simulink model "OMAP"  (R2018b)
settings: Solver=FixedStepDiscrete  StartTime=0.0  StopTime=10.0  FixedStep=0.01  RelTol=1e-3
values from neighbouring files (symbols this model uses):
  Clb_ICADirect_LaneDisp_StateFive = Simulink.Parameter    [omap_ver_442.m]
  Clb_ICADirect_LaneDisp_StateFour = Simulink.Parameter    [omap_ver_442.m]
  Clb_ICADirect_LaneDisp_StateOne = Simulink.Parameter    [omap_ver_442.m]
  Clb_ICADirect_LaneDisp_StateThree = Simulink.Parameter    [omap_ver_442.m]
  Clb_ICADirect_LaneDisp_StateTwo = Simulink.Parameter    [omap_ver_442.m]
  Clb_ICADirect_LaneDisp_StateZero = Simulink.Parameter    [omap_ver_442.m]
  Clb_ICADirect_LaneDispSW = Simulink.Parameter    [omap_ver_442.m]
  Clb_ICADirect_TrnLghtsCom_Switch = Simulink.Parameter    [omap_ver_442.m]
  Clb_ICADirect_TrnLghtsCom_Value = Simulink.Parameter    [omap_ver_442.m]
  Clb_ICADirect_TrnLghtsCrtl_Inhb = Simulink.Parameter    [omap_ver_442.m]
  OMAP_ACCAEB_EMSESC_Decel = Simulink.Parameter    [omap_ver_442.m]
  OMAP_ACCFCW_IC_Decel = Simulink.Parameter    [omap_ver_442.m]
  OMAP_clb_ACC_RVVReqType = Simulink.Parameter    [omap_ver_442.m]
  OMAP_clb_ACC_RVVReqType_Switch = Simulink.Parameter    [omap_ver_442.m]
  OMAP_clb_ACCHeadwayDisplay = Simulink.Parameter    [omap_ver_442.m]
  OMAP_clb_ACCHeadwayDisplay_Switch = Simulink.Parameter    [omap_ver_442.m]
  OMAP_clb_ACCHeadwayIcon = Simulink.Parameter    [omap_ver_442.m]
  OMAP_clb_ACCHeadwayIcon_Switch = Simulink.Parameter    [omap_ver_442.m]
  OMAP_clb_ACCMessagePrompt = Simulink.Parameter    [omap_ver_442.m]
  OMAP_clb_ACCMessagePrompt_Switch = Simulink.Parameter    [omap_ver_442.m]
  OMAP_clb_ACCRequestEPB = Simulink.Parameter    [omap_ver_442.m]
  OMAP_clb_ACCRequestEPB_Switch = Simulink.Parameter    [omap_ver_442.m]
  OMAP_clb_ACCSetSpeed = Simulink.Parameter    [omap_ver_442.m]
  OMAP_clb_ACCSetSpeed_Switch = Simulink.Parameter    [omap_ver_442.m]
  OMAP_clb_ACCSetSpeedDis = Simulink.Parameter    [omap_ver_442.m]
  OMAP_clb_ACCSetSpeedDis_Switch = Simulink.Parameter    [omap_ver_442.m]
  OMAP_clb_ACCState = Simulink.Parameter    [omap_ver_442.m]
  OMAP_clb_ACCState_Switch = Simulink.Parameter    [omap_ver_442.m]
  OMAP_clb_ACCStatusIconDis = Simulink.Parameter    [omap_ver_442.m]
  OMAP_clb_ACCStatusIconDis_Switch = Simulink.Parameter    [omap_ver_442.m]
  OMAP_clb_ACCTorqueReq = Simulink.Parameter    [omap_ver_442.m]
  OMAP_clb_ACCTorqueReq_Switch = Simulink.Parameter    [omap_ver_442.m]
  OMAP_clb_ADAS_State = Simulink.Parameter    [omap_ver_442.m]
  OMAP_clb_ADAS_State_Switch = Simulink.Parameter    [omap_ver_442.m]
  OMAP_clb_AEBAlertReq = Simulink.Parameter    [omap_ver_442.m]
  OMAP_clb_AEBAlertReq_Switch = Simulink.Parameter    [omap_ver_442.m]
  OMAP_clb_AEBBrakingProg = Simulink.Parameter    [omap_ver_442.m]
  OMAP_clb_AEBBrakingProg_Switch = Simulink.Parameter    [omap_ver_442.m]
  OMAP_clb_AEBFaultStatus = Simulink.Parameter    [omap_ver_442.m]
  OMAP_clb_AEBFaultStatus_Switch = Simulink.Parameter    [omap_ver_442.m]
  OMAP_clb_AEBMassageDisp = Simulink.Parameter    [omap_ver_442.m]
  OMAP_clb_AEBMassageDisp_Switch = Simulink.Parameter    [omap_ver_442.m]
  OMAP_clb_AEBState = Simulink.Parameter    [omap_ver_442.m]
  OMAP_clb_AEBState_Switch = Simulink.Parameter    [omap_ver_442.m]
  OMAP_clb_AEBSwitchStatus = Simulink.Parameter    [omap_ver_442.m]
  OMAP_clb_AEBSwitchStatus_Switch = Simulink.Parameter    [omap_ver_442.m]
  OMAP_clb_BrakeRequest = Simulink.Parameter    [omap_ver_442.m]
  OMAP_clb_BrakeRequest_Switch = Simulink.Parameter    [omap_ver_442.m]
  OMAP_clb_DecelerationSet = Simulink.Parameter    [omap_ver_442.m]
  OMAP_clb_DecelerationSet_Switch = Simulink.Parameter    [omap_ver_442.m]
  OMAP_clb_DecelerationType = Simulink.Parameter    [omap_ver_442.m]
  OMAP_clb_DecelerationType_Switch = Simulink.Parameter    [omap_ver_442.m]
  OMAP_clb_DeclControlReq = Simulink.Parameter    [omap_ver_442.m]
  OMAP_clb_DeclControlReq_Switch = Simulink.Parameter    [omap_ver_442.m]
  OMAP_clb_DownorUpGearMinTime = Simulink.Parameter    [omap_ver_442.m]
  OMAP_clb_DownorUpGearMinTime_Switch = Simulink.Parameter    [omap_ver_442.m]
  OMAP_clb_ELKPopupMessage = Simulink.Parameter    [omap_ver_442.m]
  OMAP_clb_ELKPopupMessage_Switch = Simulink.Parameter    [omap_ver_442.m]
  OMAP_clb_ELKSts = Simulink.Parameter    [omap_ver_442.m]
  OMAP_clb_ELKSts_Switch = Simulink.Parameter    [omap_ver_442.m]
  OMAP_clb_ESAFaultSt = Simulink.Parameter    [omap_ver_442.m]
  OMAP_clb_ESAFaultSt_Switch = Simulink.Parameter    [omap_ver_442.m]
  OMAP_clb_ESARequest = Simulink.Parameter    [omap_ver_442.m]
  OMAP_clb_ESARequest_Switch = Simulink.Parameter    [omap_ver_442.m]
  OMAP_clb_ESAState = Simulink.Parameter    [omap_ver_442.m]
  OMAP_clb_ESAState_Switch = Simulink.Parameter    [omap_ver_442.m]
  OMAP_clb_ESATorqueReq = Simulink.Parameter    [omap_ver_442.m]
  OMAP_clb_ESATorqueReq_Switch = Simulink.Parameter    [omap_ver_442.m]
  OMAP_clb_ESCDriveOff = Simulink.Parameter    [omap_ver_442.m]
  OMAP_clb_ESCDriveOff_Switch = Simulink.Parameter    [omap_ver_442.m]
  OMAP_clb_ESCHoldReq = Simulink.Parameter    [omap_ver_442.m]
  OMAP_clb_ESCHoldReq_Switch = Simulink.Parameter    [omap_ver_442.m]
  OMAP_clb_Handsoffwarning = Simulink.Parameter    [omap_ver_442.m]
  OMAP_clb_Handsoffwarning_Switch = Simulink.Parameter    [omap_ver_442.m]
  OMAP_clb_HapticAlarmReq = Simulink.Parameter    [omap_ver_442.m]
  OMAP_clb_HapticAlarmReq_Switch = Simulink.Parameter    [omap_ver_442.m]
  OMAP_clb_HMIPopupMassage = Simulink.Parameter    [omap_ver_442.m]
  OMAP_clb_HMIPopupMassage_Switch = Simulink.Parameter    [omap_ver_442.m]
  OMAP_clb_HWAActionSts = Simulink.Parameter    [omap_ver_442.m]
  OMAP_clb_HWAActionSts_Switch = Simulink.Parameter    [omap_ver_442.m]
  OMAP_clb_HWAMode = Simulink.Parameter    [omap_ver_442.m]
  OMAP_clb_HWAMode_Switch = Simulink.Parameter    [omap_ver_442.m]
  OMAP_clb_HWATurnOnIdctr = Simulink.Parameter    [omap_ver_442.m]
  OMAP_clb_HWATurnOnIdctr_Switch = Simulink.Parameter    [omap_ver_442.m]
  OMAP_clb_ICAMassageDisp = Simulink.Parameter    [omap_ver_442.m]
  OMAP_clb_ICAMassageDisp_Switch = Simulink.Parameter    [omap_ver_442.m]
  OMAP_clb_ICAStatusIcon = Simulink.Parameter    [omap_ver_442.m]
  OMAP_clb_ICAStatusIcon_Switch = Simulink.Parameter    [omap_ver_442.m]
  OMAP_clb_ISLCDriverRemind = Simulink.Parameter    [omap_ver_442.m]
  OMAP_clb_ISLCDriverRemind_Switch = Simulink.Parameter    [omap_ver_442.m]
  OMAP_clb_ISLCState = Simulink.Parameter    [omap_ver_442.m]
  OMAP_clb_ISLCState_Switch = Simulink.Parameter    [omap_ver_442.m]
  OMAP_clb_JAFaultSt = Simulink.Parameter    [omap_ver_442.m]
  OMAP_clb_JAFaultSt_Switch = Simulink.Parameter    [omap_ver_442.m]
  OMAP_clb_LCAPopupMessage = Simulink.Parameter    [omap_ver_442.m]
  OMAP_clb_LCAPopupMessage_Switch = Simulink.Parameter    [omap_ver_442.m]
  OMAP_clb_LCAStatusDisplay = Simulink.Parameter    [omap_ver_442.m]
  OMAP_clb_LCAStatusDisplay_Switch = Simulink.Parameter    [omap_ver_442.m]
  OMAP_clb_LDWStatusDisplay = Simulink.Parameter    [omap_ver_442.m]
  OMAP_clb_LDWStatusDisplay_Switch = Simulink.Parameter    [omap_ver_442.m]
  OMAP_clb_LDWWarningSt = Simulink.Parameter    [omap_ver_442.m]
  OMAP_clb_LDWWarningSt_Switch = Simulink.Parameter    [omap_ver_442.m]
  OMAP_clb_LightControlValid = Simulink.Parameter    [omap_ver_442.m]
  OMAP_clb_LightControlValid_Switch = Simulink.Parameter    [omap_ver_442.m]
  OMAP_clb_LKAActivation = Simulink.Parameter    [omap_ver_442.m]
  OMAP_clb_LKAActivation_Switch = Simulink.Parameter    [omap_ver_442.m]
  OMAP_clb_LKAAngleReq = Simulink.Parameter    [omap_ver_442.m]
  OMAP_clb_LKAAngleReq_Switch = Simulink.Parameter    [omap_ver_442.m]
  OMAP_clb_LKAMode = Simulink.Parameter    [omap_ver_442.m]
  OMAP_clb_LKAMode_Switch = Simulink.Parameter    [omap_ver_442.m]
  OMAP_clb_LKAorELK_CoolTime = Simulink.Parameter    [omap_ver_442.m]
  OMAP_clb_LKAState = Simulink.Parameter    [omap_ver_442.m]
  OMAP_clb_LKAState_Switch = Simulink.Parameter    [omap_ver_442.m]
  OMAP_clb_LKAStatusDisplay = Simulink.Parameter    [omap_ver_442.m]
  OMAP_clb_LKAStatusDisplay_Switch = Simulink.Parameter    [omap_ver_442.m]
  OMAP_clb_LKASwitchState = Simulink.Parameter    [omap_ver_442.m]
  OMAP_clb_LKASwitchState_Switch = Simulink.Parameter    [omap_ver_442.m]
  OMAP_clb_LKATorqFactReq = Simulink.Parameter    [omap_ver_442.m]
  OMAP_clb_LKATorqFactReq_Switch = Simulink.Parameter    [omap_ver_442.m]
  OMAP_clb_PrefillRequest = Simulink.Parameter    [omap_ver_442.m]
  ... (+36 more)
libraries: simulink x184, canmsglib x2
(part 10 of 14)

== system OMAP/Runnable_OMAP_10ms_sys/OMAP_Module/ICA_Direct_G59/ICA_Define/Subsystem1/Dspl ==
  note: 0是运动，1是静止
  note: 0 ：可以从降级回到正常，
      | 1 ：不可以从降级回到正常
  TxHndOff : Inport
  Dspl_stTkOvStChk : Inport  Port=2
  Dspl_facmL0Ql : Inport  Port=3
  Dspl_facmR0Ql : Inport  Port=4
  Dspl_stVehSty : Inport  Port=5
  Dspl_facmL0Type : Inport  Port=6
  Dspl_facmR0Type : Inport  Port=7
  Dspl_stTHState : Inport  Port=8
  Dspl_bsFromFMCMsg : Inport  Port=9
  Dspl_stTHFKeyState : Inport  Port=10
  DsplPrcs_CIb : Inport  Port=11
  Dspl_tfAddVocCmd : Inport  Port=12
  DsplPrcs_dDgrdIconWarnflag : Inport  Port=13
  DsplPrcs_stSWALimFlg : Inport  Port=14
  Dspl_stturn_lightState : Inport  Port=15
  Dspl_stTLC_ALCmodeSW : Inport  Port=16
  Dspl_stLC_SpdCndtFlg : Inport  Port=17
  Bus Selector5 : BusSelector  OutputSignals=TH_HMIClb_tiHndOffTxtWarnT_C,TH_HMIClb_tiDgrdVocWarnDurT_C,TH_HMIClb_tiHndOffVocWarnT_C,TH_HMIClb_tiTxtLimT_C,TH_HMIClb_tiDgrdIconWarnHiDurT_C,TH_HMIClb_tiDgrdIconWarnLoDurT_C,TH_HMIClb_tiSWALimFlgDetT_C,TH_HMIClb_tiCalcPer_C
  Data Type Conversion{,1..6} (7 alike) : DataTypeConversion  OutDataTypeStr=uint16
  DsplPrcs : Subsystem
  TimePrcs : Subsystem
  Dspl_stTxtDspl : Outport
  Dspl_stICAIcon : Outport  Port=2
  Dspl_stLaneDspl : Outport  Port=3
  Dspl_stL0DispType : Outport  Port=4
  Dspl_stR0DispType : Outport  Port=5
  Dspl_stVocDspl : Outport  Port=6
  Dspl_stHWAmode : Outport  Port=7
  Dspl_bsMon : Outport  Port=8
  wires:
  Dspl_stTHState/1 -> DsplPrcs/7(DsplPrcs_stTHState)
  Dspl_stTHFKeyState/1 -> DsplPrcs/9(DsplPrcs_stTHFKeyState)
  Dspl_bsFromFMCMsg/1 -> DsplPrcs/8(DsplPrcs_bsFromFMCMsg)
  Data Type Conversion/1 -> Dspl_stTxtDspl/1
  Data Type Conversion1/1 -> Dspl_stICAIcon/1
  Data Type Conversion2/1 -> Dspl_stLaneDspl/1
  DsplPrcs/6(DsplPrcs_stVocDspl) -> Data Type Conversion5/1
  DsplPrcs/1(DsplPrcs_stTxtDspl) -> Data Type Conversion/1
  DsplPrcs/2(DsplPrcs_stICAIcon) -> Data Type Conversion1/1
  Data Type Conversion5/1 -> Dspl_stVocDspl/1
  DsplPrcs/8(DsplPrcs_bsMon) -> Dspl_bsMon/1
  DsplPrcs_CIb/1 -> Bus Selector5/1
  TimePrcs/2(TimePrcs_dDgrdVocWarnDurnum) -> DsplPrcs/18(DsplPrcs_dDgrdVocWarnDurnum)
  TimePrcs/3(TimePrcs_dHndOffVocWarnnum) -> DsplPrcs/19(DsplPrcs_dHndOffVocWarnnum)
  TimePrcs/1(TimePrcs_dHndOffTxtWarnnum) -> DsplPrcs/17(DsplPrcs_dHndOffTxtWarnnum)
  TimePrcs/4(TimePrcs_dTxtLimnum) -> DsplPrcs/20(DsplPrcs_dTxtLimnum)
  Bus Selector5/3 -> TimePrcs/3(TimePrcs_tiHndOffVocWarnT_C)  "<TH_HMIClb_tiHndOffVocWarnT_C>"
  Bus Selector5/8 -> TimePrcs/8(TimePrcs_tiCalcPer_C)  "<TH_HMIClb_tiCalcPer_C>"
  Bus Selector5/4 -> TimePrcs/4(TimePrcs_tiTxtLimT_C)  "<TH_HMIClb_tiTxtLimT_C>"
  Bus Selector5/1 -> TimePrcs/1(TimePrcs_tiHndOffTxtWarnT_C)  "<TH_HMIClb_tiHndOffTxtWarnT_C>"
  Bus Selector5/2 -> TimePrcs/2(TimePrcs_tiDgrdVocWarnDurT_C)  "<TH_HMIClb_tiDgrdVocWarnDurT_C>"
  TxHndOff/1 -> DsplPrcs/1(DsplPrcs_stStWhlHld)
  Dspl_facmL0Ql/1 -> DsplPrcs/3(DsplPrcs_facmL0Ql)
  Dspl_facmR0Ql/1 -> DsplPrcs/4(DsplPrcs_facmR0Ql)
  Dspl_stVehSty/1 -> DsplPrcs/10(DsplPrcs_stVehSty)
  Dspl_tfAddVocCmd/1 -> DsplPrcs/11(DsplPrcs_tfAddVocCmd)
  TimePrcs/5(TimePrcs_dDgrdIconWarnHiDurnum) -> DsplPrcs/21(DsplPrcs_dDgrdIconWarnHiDurnum)
  TimePrcs/6(TimePrcs_dDgrdIconWarnLoDurnum) -> DsplPrcs/22(DsplPrcs_dDgrdIconWarnLoDurnum)
  Bus Selector5/5 -> TimePrcs/5(TimePrcs_tiDgrdIconWarnHiDurT_C)  "<TH_HMIClb_tiDgrdIconWarnHiDurT_C>"
  Bus Selector5/6 -> TimePrcs/6(TimePrcs_tiDgrdIconWarnLoDurT_C)  "<TH_HMIClb_tiDgrdIconWarnLoDurT_C>"
  DsplPrcs_dDgrdIconWarnflag/1 -> DsplPrcs/13(DsplPrcs_dDgrdIconWarnflag)
  DsplPrcs_stSWALimFlg/1 -> DsplPrcs/12(DsplPrcs_stSWALimFlg)
  Bus Selector5/7 -> TimePrcs/7(TimePrcs_tiSWALimFlgDetT_C)  "<TH_HMIClb_tiSWALimFlgDetT_C>"
  TimePrcs/7(TimePrcs_tiSWALimFlgDetnum) -> DsplPrcs/23(DsplPrcs_tiSWALimFlgDetnum)
  Dspl_stTkOvStChk/1 -> DsplPrcs/2(DsplPrcs_stTkOvStChk)
  Dspl_facmL0Type/1 -> DsplPrcs/5(DsplPrcs_facmL0Type)
  Dspl_facmR0Type/1 -> DsplPrcs/6(DsplPrcs_facmR0Type)
  Data Type Conversion3/1 -> Dspl_stL0DispType/1
  Data Type Conversion4/1 -> Dspl_stR0DispType/1
  DsplPrcs/3(DsplPrcs_stLaneDspl) -> Data Type Conversion2/1
  DsplPrcs/4(DsplPrcs_stL0DispType) -> Data Type Conversion3/1
  DsplPrcs/5(DsplPrcs_stR0DispType) -> Data Type Conversion4/1
  Dspl_stturn_lightState/1 -> DsplPrcs/14(DsplPrcs_stturn_lightState)
  Dspl_stTLC_ALCmodeSW/1 -> DsplPrcs/15(DsplPrcs_stTLC_ALCmodeSW)
  Dspl_stLC_SpdCndtFlg/1 -> DsplPrcs/16(DsplPrcs_stLC_SpdCndtFlg)
  DsplPrcs/7(DsplPrcs_stHWAmode) -> Data Type Conversion6/1
  Data Type Conversion6/1 -> Dspl_stHWAmode/1

== system OMAP/Runnable_OMAP_10ms_sys/OMAP_Module/ICA_Direct_G59/ICA_Define/Subsystem1/Subsystem ==
  Vehicle_Line_Display_Org : Inport
  LCRMode : Inport  Port=2
  High_Time : Inport  Port=3
  Low_Time : Inport  Port=4
  ISA_Value : Inport  Port=5
  ISA_Type : Inport  Port=6
  THMode : Inport  Port=7
  LC_Scene : Inport  Port=8
  Compare To Constant : simulink/Logic and Bit Operations/Compare To Constant  relop===  const=uint16(4)  OutDataTypeStr=boolean
  Compare To Constant1 : simulink/Logic and Bit Operations/Compare To Constant  relop===  const=uint16(2)  OutDataTypeStr=boolean
  Compare To Constant2 : simulink/Logic and Bit Operations/Compare To Constant  relop===  const=uint16(3)  OutDataTypeStr=boolean
  Constant4 : Constant  Value=0  OutDataTypeStr=uint16
  Constant5 : Constant  Value=0  OutDataTypeStr=uint16
  Constant6 : Constant  Value=0  OutDataTypeStr=uint16
  Data Type Conversion : DataTypeConversion  OutDataTypeStr=uint16
  Data Type Conversion1 : DataTypeConversion  OutDataTypeStr=uint16
  Gain : Gain  Gain=100
  Gain1 : Gain  Gain=100
  Logical Operator1 : Logic  Operator=OR  AllPortsSameDT=off  OutDataTypeStr=boolean
  MATLAB Function : MATLAB Function  TreatAsAtomicUnit=on
  Subsystem : Subsystem
  Switch{1..3,6} (4 alike) : Switch  Criteria=u2 > Threshold
  TSR_Version_Only_Sign_Type : Outport
  Vehicle_Line_Display : Outport  Port=2
  ISA Value : Outport  Port=3
  wires:
  Vehicle_Line_Display_Org/1 -> Vehicle_Line_Display/1
  Compare To Constant/1 -> Switch1/2
  MATLAB Function/1(TSR_Version_Only_Sign_Type) -> Switch2/1, Switch1/1
  Switch1/1 -> TSR_Version_Only_Sign_Type/1
  Subsystem/1(Signal) -> Switch2/2
  Constant5/1 -> Switch2/3
  Switch2/1 -> Switch3/1
  Constant6/1 -> Switch3/3
  Switch3/1 -> Switch1/3
  Logical Operator1/1 -> Switch3/2
  High_Time/1 -> Gain/1
  Low_Time/1 -> Gain1/1
  Gain/1 -> Data Type Conversion/1
  Gain1/1 -> Data Type Conversion1/1
  Data Type Conversion/1 -> Subsystem/1(HiDurnum)
  Data Type Conversion1/1 -> Subsystem/2(LoDurnum)
  THMode/1 -> [THMode], Compare To Constant/1
  ISA_Value/1 -> Switch6/1, Switch6/2
  Constant4/1 -> Switch6/3
  Switch6/1 -> ISA Value/1
  LC_Scene/1 -> MATLAB Function/2(LC_Scene)
  [THMode] -> MATLAB Function/1(TH_Mode)
  LCRMode/1 -> [stLCRMode], Compare To Constant1/1, Compare To Constant2/1
  Compare To Constant1/1 -> Logical Operator1/1
  Compare To Constant2/1 -> Logical Operator1/2
  [stLCRMode] -> MATLAB Function/3(stLCRMode)

== system OMAP/Runnable_OMAP_10ms_sys/OMAP_Module/ICA_Direct_G59/ICA_Define/Subsystem1/Subsystem1 ==
  note: 标定开关Calib_ICADirect_TrnLghtsCom_Switch默认值为1，走ICA_Direct内部判断
      | 标定值为0时，通过标定值Calib_ICADirect_TrnLghtsCom_Value来自主选择输出的值
  LCRMode : Inport
  Constant : Constant  OutDataTypeStr=uint16
  Constant1 : Constant  Value=2  OutDataTypeStr=uint16
  Constant2 : Constant  Value=0  OutDataTypeStr=uint16
  Constant3 : Constant  Value=Clb_ICADirect_TrnLghtsCom_Switch  OutDataTypeStr=uint16
  Constant4 : Constant  Value=Clb_ICADirect_TrnLghtsCom_Value  OutDataTypeStr=uint16
  Index Vector : MultiPortSwitch  DataPortOrder=Specify indices  DataPortIndices={2,3,0}  OutDataTypeStr=uint16
  Switch : Switch  Criteria=u2 > Threshold  OutDataTypeStr=uint16
  TurnLightsCmd : Outport
  wires:
  LCRMode/1 -> Index Vector/1
  Index Vector/1 -> Switch/1
  Constant/1 -> Index Vector/2
  Constant1/1 -> Index Vector/3
  Constant2/1 -> Index Vector/4
  Constant3/1 -> Switch/2
  Constant4/1 -> Switch/3
  Switch/1 -> TurnLightsCmd/1

== system OMAP/Runnable_OMAP_10ms_sys/OMAP_Module/ICA_Direct_G59/ICA_Define/TH_HMIClb/ISA_TYPE ==
  In2 : Inport
  Switch : Switch  Criteria=u2 ~= 0  OutDataTypeStr=uint16
  tmp : Constant  Value=0  OutDataTypeStr=uint16
  Out1 : Outport
  wires:
  In2/1 -> Switch/2, Switch/1
  Switch/1 -> Out1/1
  tmp/1 -> Switch/3

== system OMAP/Runnable_OMAP_10ms_sys/OMAP_Module/ICA_Direct_G59/ICA_Define/TH_HMIClb/ISA_Value ==
  In2 : Inport
  Switch : Switch  Criteria=u2 ~= 0  OutDataTypeStr=uint16
  tmp : Constant  Value=0  OutDataTypeStr=uint16
  Out1 : Outport
  wires:
  tmp/1 -> Switch/3
  Switch/1 -> Out1/1
  In2/1 -> Switch/1, Switch/2

== system OMAP/Runnable_OMAP_10ms_sys/OMAP_Module/ICA_Direct_G59/ICA_Define/TH_HMIClb/LCScene_tmp ==
  In2 : Inport
  Switch : Switch  Criteria=u2 ~= 0  OutDataTypeStr=uint16
  tmp : Constant  Value=0  OutDataTypeStr=uint16
  Out1 : Outport
  wires:
  In2/1 -> Switch/2, Switch/1
  Switch/1 -> Out1/1
  tmp/1 -> Switch/3

== system OMAP/Runnable_OMAP_10ms_sys/OMAP_Module/ICA_Direct_G59/ICA_Define/TH_HMIClb/Mode_tmp ==
  In2 : Inport
  Switch : Switch  Criteria=u2 ~= 0  OutDataTypeStr=uint16
  tmp : Constant  Value=0  OutDataTypeStr=uint16
  Out1 : Outport
  wires:
  tmp/1 -> Switch/3
  Switch/1 -> Out1/1
  In2/1 -> Switch/1, Switch/2

== system OMAP/Runnable_OMAP_10ms_sys/OMAP_Module/ICA_Direct_G59/ICA_Define/TH_HMIClb/TH_HMIClb_tiDgrdIconWarnHiDurT_C ==
  In2 : Inport
  Constant : Constant  Value=TH_HMIClb_tiDgrdIconWarnHiDurT_C  OutDataTypeStr=single
  Switch : Switch  Criteria=u2 ~= 0  OutDataTypeStr=single
  Out1 : Outport
  wires:
  Constant/1 -> Switch/3
  Switch/1 -> Out1/1
  In2/1 -> Switch/1, Switch/2

== system OMAP/Runnable_OMAP_10ms_sys/OMAP_Module/ICA_Direct_G59/ICA_Define/TH_HMIClb/TH_HMIClb_tiDgrdIconWarnLoDurT_C ==
  In2 : Inport
  Constant : Constant  Value=TH_HMIClb_tiDgrdIconWarnLoDurT_C  OutDataTypeStr=single
  Switch : Switch  Criteria=u2 ~= 0  OutDataTypeStr=single
  Out1 : Outport
  wires:
  In2/1 -> Switch/2, Switch/1
  Switch/1 -> Out1/1
  Constant/1 -> Switch/3

== system OMAP/Runnable_OMAP_10ms_sys/OMAP_Module/ICA_Direct_G59/ICA_Define/TH_HMIClb/TH_HMIClb_tiDgrdVocWarnDurT_C ==
  In2 : Inport
  Switch : Switch  Criteria=u2 ~= 0  OutDataTypeStr=single
  TH_MIN_SPEED_UPPER 1 : Constant  Value=TH_HMIClb_tiDgrdVocWarnDurT_C  OutDataTypeStr=single
  Out1 : Outport
  wires:
  In2/1 -> Switch/2, Switch/1
  Switch/1 -> Out1/1
  TH_MIN_SPEED_UPPER 1/1 -> Switch/3

== system OMAP/Runnable_OMAP_10ms_sys/OMAP_Module/ICA_Direct_G59/ICA_Define/TH_HMIClb/TH_HMIClb_tiHndOffTxtWarnT_C  ==
  In2 : Inport
  Switch : Switch  Criteria=u2 ~= 0  OutDataTypeStr=single
  TH_MIN_SPEED_UPPER 1 : Constant  Value=TH_HMIClb_tiHndOffTxtWarnT_C  OutDataTypeStr=single
  Out1 : Outport
  wires:
  In2/1 -> Switch/2, Switch/1
  Switch/1 -> Out1/1
  TH_MIN_SPEED_UPPER 1/1 -> Switch/3

== system OMAP/Runnable_OMAP_10ms_sys/OMAP_Module/ICA_Direct_G59/ICA_Define/TH_HMIClb/TH_HMIClb_tiHndOffVocWarnT_C ==
  In2 : Inport
  Switch : Switch  Criteria=u2 ~= 0  OutDataTypeStr=single
  TH_MIN_SPEED_UPPER 1 : Constant  Value=TH_HMIClb_tiHndOffVocWarnT_C  OutDataTypeStr=single
  Out1 : Outport
  wires:
  TH_MIN_SPEED_UPPER 1/1 -> Switch/3
  Switch/1 -> Out1/1
  In2/1 -> Switch/1, Switch/2

== system OMAP/Runnable_OMAP_10ms_sys/OMAP_Module/ICA_Direct_G59/ICA_Define/TH_HMIClb/TH_HMIClb_tiSWALimFlgDetT_C ==
  In2 : Inport
  Switch : Switch  Criteria=u2 ~= 0  OutDataTypeStr=single
  TH_HMIClb_tiSWALimFlgDetT_C : Constant  Value=TH_HMIClb_tiSWALimFlgDetT_C  OutDataTypeStr=single
  Out1 : Outport
  wires:
  TH_HMIClb_tiSWALimFlgDetT_C/1 -> Switch/3
  Switch/1 -> Out1/1
  In2/1 -> Switch/1, Switch/2

== system OMAP/Runnable_OMAP_10ms_sys/OMAP_Module/ICA_Direct_G59/ICA_Define/TH_HMIClb/TH_HMIClb_tiTxtLimT_C ==
  In2 : Inport
  Constant : Constant  Value=TH_HMIClb_tiTxtLimT_C  OutDataTypeStr=single
  Switch : Switch  Criteria=u2 ~= 0  OutDataTypeStr=single
  Out1 : Outport
  wires:
  In2/1 -> Switch/2, Switch/1
  Switch/1 -> Out1/1
  Constant/1 -> Switch/3

== system OMAP/Runnable_OMAP_10ms_sys/OMAP_Module/Subsystem/EMS_Arbitration/ACC//ICA_arb_AEB//JA/AEB_arb_JA ==
  note: 仲裁#1——AEB与JA
      | 1. JAEB/JACW无条件优先于FCW
      | 2. （在AEB系统内部，已经是AEB无条件优先于FCW）
      | 3. 对于AEB和JAEB/JACW，使能请求取或，请求值取较大者（若JA只开启报警、未开启制动，也就是只有JACW，那么制动请求值就很小，同样能符合此条效果）
      | 4. AEB_Alert能够标记减速发送者：2（AEB制动）、3（JA制动）
  Input_AEBS : Inport
  Input_JABS : Inport  Port=2
  Bus Creator3 : BusCreator  Inputs=5
  Bus Selector : BusSelector  OutputSignals=AEBSve_d_MDDdecRequest_convert,AEBSve_g_DecSetpoint_convert
  Bus Selector4 : BusSelector  OutputSignals=JABSve_d_DbMDDdecRequest_convert
  Compare To Constant1 : simulink/Logic and Bit Operations/Compare To Constant  relop=<  const=-2  OutDataTypeStr=boolean
  Compare To Constant4 : simulink/Logic and Bit Operations/Compare To Constant  relop===  const=1  OutDataTypeStr=boolean
  Compare To Constant5 : simulink/Logic and Bit Operations/Compare To Constant  relop===  const=1  OutDataTypeStr=boolean
  Compare To Constant6 : simulink/Logic and Bit Operations/Compare To Constant  relop=>=  const=-2  OutDataTypeStr=boolean
  Compare To Constant9 : simulink/Logic and Bit Operations/Compare To Constant  relop===  const=1  OutDataTypeStr=boolean
  Logical Operator : Logic  Operator=OR  AllPortsSameDT=off  OutDataTypeStr=boolean
  Logical Operator2 : Logic  AllPortsSameDT=off  OutDataTypeStr=boolean
  Logical Operator3 : Logic  AllPortsSameDT=off  OutDataTypeStr=boolean
  OMAPve_g_ACCTqReqNum1 : Constant  Value=-4000  OutDataTypeStr=single
  OMAPve_g_PotACCTqReqNum1 : Constant  Value=-4000  OutDataTypeStr=single
  OMAPve_g_TminUp_or_downGearNum2 : Constant  Value=0  OutDataTypeStr=single
  OMAPve_y_Powertrain_torquewheel_requestNum1 : Constant  Value=0  OutDataTypeStr=uint8
  OMAPve_y_stAcvTqWhlPTPotReqNum2 : Constant  Value=2  OutDataTypeStr=uint8
  Out1 : Outport
  Out2 : Outport  Port=2
  Out3 : Outport  Port=3
  wires:
  OMAPve_g_ACCTqReqNum1/1 -> Bus Creator3/2  "OMAPve_g_ACCTqReq_1"
  Compare To Constant9/1 -> Logical Operator2/1
  Input_AEBS/1 -> Bus Selector/1
  Bus Creator3/1 -> Out1/1
  OMAPve_g_PotACCTqReqNum1/1 -> Bus Creator3/1  "OMAPve_g_PotACCTqReq_1"
  OMAPve_g_TminUp_or_downGearNum2/1 -> Bus Creator3/4  "OMAPve_g_TminUp_or_downGear_1"
  Logical Operator2/1 -> Out3/1
  Compare To Constant4/1 -> Logical Operator/2
  OMAPve_y_stAcvTqWhlPTPotReqNum2/1 -> Bus Creator3/5  "OMAPve_y_stAcvTqWhlPTPotReq_1"
  Input_JABS/1 -> Bus Selector4/1
  Compare To Constant1/1 -> Logical Operator3/2
  OMAPve_y_Powertrain_torquewheel_requestNum1/1 -> Bus Creator3/3  "OMAPve_y_Powertrain_torquewheel_request_1"
  Bus Selector/1 -> Compare To Constant5/1, Compare To Constant9/1  "<AEBSve_d_MDDdecRequest_convert>"
  Bus Selector4/1 -> Compare To Constant4/1  "<JABSve_d_DbMDDdecRequest_convert>"
  Logical Operator/1 -> Out2/1
  Bus Selector/2 -> Compare To Constant1/1, Compare To Constant6/1  "<AEBSve_g_DecSetpoint_convert>"
  Compare To Constant6/1 -> Logical Operator2/2
  Logical Operator3/1 -> Logical Operator/1
  Compare To Constant5/1 -> Logical Operator3/1

== system OMAP/Runnable_OMAP_10ms_sys/OMAP_Module/Subsystem/EPS_Default_Arbitration/LKA_arb_ELK/Subsystem ==
  LKA_State : Inport
  ELK_State : Inport  Port=2
  In1 : Inport  Port=3
  Compare To Constant1 : simulink/Logic and Bit Operations/Compare To Constant  relop===  const=4  OutDataTypeStr=boolean
  Compare To Constant2 : simulink/Logic and Bit Operations/Compare To Constant  relop===  const=4  OutDataTypeStr=boolean
  Logical Operator : Logic  AllPortsSameDT=off  OutDataTypeStr=boolean
  Logical Operator1 : Logic  AllPortsSameDT=off  OutDataTypeStr=boolean
  Logical Operator2 : Logic  Operator=OR  AllPortsSameDT=off  OutDataTypeStr=boolean
  Logical Operator3 : Logic  Operator=OR  AllPortsSameDT=off  OutDataTypeStr=boolean
  Logical Operator4 : Logic  Operator=NOT  AllPortsSameDT=off  OutDataTypeStr=boolean
  Logical Operator5 : Logic  Operator=OR  AllPortsSameDT=off  OutDataTypeStr=boolean
  Memory : Memory
  Subsystem1 : Subsystem
  Subsystem2 : Subsystem
  Switch : Switch  Criteria=u2 > Threshold
  Out1 : Outport
  wires:
  Logical Operator1/1 -> Logical Operator5/2
  Logical Operator/1 -> Logical Operator5/1
  Logical Operator5/1 -> Switch/2, Memory/1
  Memory/1 -> Logical Operator1/2
  Subsystem2/1(Out1) -> Logical Operator1/1, Logical Operator2/2
  LKA_State/1 -> Compare To Constant2/1, Switch/3
  ELK_State/1 -> Switch/1, Compare To Constant1/1
  Compare To Constant1/1 -> Logical Operator2/1, Subsystem2/1(In1)
  Switch/1 -> Out1/1
  Compare To Constant2/1 -> Subsystem1/1(In1), Logical Operator3/1
  Subsystem1/1(Out1) -> Logical Operator3/2
  In1/1 -> Subsystem1/2(In2), Subsystem2/2(In2)
  Logical Operator2/1 -> Logical Operator/1
  Logical Operator3/1 -> Logical Operator4/1
  Logical Operator4/1 -> Logical Operator/2

== system OMAP/Runnable_OMAP_10ms_sys/OMAP_Module/Subsystem/EPS_Default_Arbitration/LKA_arb_ELK/Subsystem2 ==
  <LKASve_y_EPS_State_Control_convert> : Inport
  <OMAPve_y_General_state_of_LKA_function3F2_2> : Inport  Port=2
  Chart1 : Stateflow chart  TreatAsAtomicUnit=on
  Constant : Constant  Value=OMAP_clb_LKAorELK_CoolTime  OutDataTypeStr=single
  Subsystem1 : Subsystem
  state : Outport
  wires:
  Subsystem1/6(ELK_Active) -> Chart1/6(ELK_Active)
  Subsystem1/2(LKA_Down) -> Chart1/2(LKA_Down)
  Subsystem1/1(LKA_Up) -> Chart1/1(LKA_Up)
  Subsystem1/3(LKA_Active) -> Chart1/3(LKA_Active)
  <OMAPve_y_General_state_of_LKA_function3F2_2>/1 -> Subsystem1/2(ELK_State)
  <LKASve_y_EPS_State_Control_convert>/1 -> Subsystem1/1(LKA_State)
  Subsystem1/4(ELK_Up) -> Chart1/4(ELK_Up)
  Subsystem1/5(ELK_Down) -> Chart1/5(ELK_Down)
  Constant/1 -> Chart1/7(cool_time)
  Chart1/1(state) -> state/1

== system OMAP/Runnable_OMAP_10ms_sys/OMAP_Module/Subsystem/ESC_Arbitration/ACC//ICA_arb_AEB//JA/AEB_arb_JA ==
  note: 仲裁#1——AEB与JA
      | 1. JAEB/JACW无条件优先于FCW
      | 2. （在AEB系统内部，已经是AEB无条件优先于FCW）
      | 3. 对于AEB和JAEB/JACW，使能请求取或，请求值取较大者（若JA只开启报警、未开启制动，也就是只有JACW，那么制动请求值就很小，同样能符合此条效果）
      | 4. AEB_Alert能够标记减速发送者：2（AEB制动）、3（JA制动）
  note: 仲裁#11——AEB与JA的STATUS
      | 1. 关于对执行器发出的AEB_STATE——
      | 值7：对内，各自判断、各自对自己生效；对外OMAP发送：任一方fault就fault
      | 值6、5：对内，各自判断、各自对自己生效；对外OMAP发送：只以AEB的为准。特殊情况：如果AEB在3，但是JA在6、5，则对外发6、5
      | 值4：不用
      | 值3：对内，各自判断、各自对自己生效；对外OMAP发送：双方都inhibit才inhibit
      | 值2：不用
      | 值1：对内：JA可以不做。对外OMAP发送：只以AEB的为准
      | 值0：对内：JA可以不做。对外OMAP发送：只以AEB的为准
  note: 仲裁#8——AEB/FCW/JAEB/JACW与ELK
      | 1.AEB/FCW/JAEB/JACW无条件优先于ELK
  Input_AEBS : Inport
  Input_JABS : Inport  Port=2
  Input_ELKS : Inport  Port=3
  AEB/JA_arb_ELK : Subsystem
  AEB_arb_JA_STATUS : Subsystem
  Bus Creator : BusCreator  Inputs=5
  Bus Creator1 : BusCreator  Inputs=8
  Bus Selector5 : BusSelector  OutputSignals=AEBSve_d_FCWStatus_convert,AEBSve_d_functionFARCState_convert,AEBSve_d_AEBStatus_convert,AEBSve_d_Prefill_request_convert,AEBSve_d_AEBAlertReq_convert,AEBSve_d_HapticAlarm_convert,AEBSve_d_ESCDriveOff_convert,AEBSve_d_ESCHoldReq_convert,AEBSve_d_MDDdecType_convert,AEBSve_d_Braking_progress_convert,AEBSve_d_MDDdecRequest_convert,AEBSve_g_DecSetpoint_convert
  Bus Selector6 : BusSelector  OutputSignals=JABSve_g_DbDecSetpoint_convert,JABSve_d_DbMDDdecType_convert,JABSve_d_DbMDDdecRequest_convert,JABSve_d_DbPrefillReq_convert,JABSve_d_DbAlertReq_convert,JABSve_d_DbHapticAlarm_convert,JABSve_d_DbESCDriveOff_convert,JABSve_d_DbESCHoldReq_convert,JABSve_d_DbFunFARCSta_convert,JABSve_d_DbJACWStatus_convert
  Compare To Constant3 : simulink/Logic and Bit Operations/Compare To Constant  relop=<  const=-2  OutDataTypeStr=boolean
  Compare To Constant4 : simulink/Logic and Bit Operations/Compare To Constant  relop===  const=1  OutDataTypeStr=boolean
  Compare To Constant5 : simulink/Logic and Bit Operations/Compare To Constant  relop===  const=1  OutDataTypeStr=boolean
  Compare To Constant7 : simulink/Logic and Bit Operations/Compare To Constant  relop=>=  const=-2  OutDataTypeStr=boolean
  Compare To Constant8 : simulink/Logic and Bit Operations/Compare To Constant  relop===  const=1  OutDataTypeStr=boolean
  Data Type Conversion{1..2,9..10} (4 alike) : DataTypeConversion  OutDataTypeStr=uint8
  Logical Operator{,1,7..9} (5 alike) : Logic  Operator=OR  AllPortsSameDT=off  OutDataTypeStr=boolean
  Logical Operator2 : Logic  AllPortsSameDT=off  OutDataTypeStr=boolean
  Logical Operator5 : Logic  AllPortsSameDT=off  OutDataTypeStr=boolean
  OMAPve_y_ADAS_ACCRequestEPBNum : Constant  Value=0  OutDataTypeStr=uint8
  Relational Operator : RelationalOperator  Operator=<=  OutDataTypeStr=boolean  RndMeth=Simplest
  Switch10 : Switch  Criteria=u2 ~= 0  OutDataTypeStr=single
  Switch3 : Switch  Criteria=u2 ~= 0  OutDataTypeStr=uint8
  Switch6 : Switch  Criteria=u2 ~= 0  OutDataTypeStr=uint8
  Switch9 : Switch  Criteria=u2 ~= 0  OutDataTypeStr=uint8
  Terminator : Terminator
  Out1 : Outport
  Out2 : Outport  Port=2
  Out3 : Outport  Port=3
  Out4 : Outport  Port=4
  tag scope: ob_AEBarbJADecReq=global, ob_AEBarbJADecSet=global, ob_AEBarbJADecType=global
  wires:
  Bus Selector5/3 -> Terminator/1  "<AEBSve_d_AEBStatus_convert>"
  Bus Selector6/1 -> Switch10/3, Relational Operator/2  "<JABSve_g_DbDecSetpoint_convert>"
  Input_JABS/1 -> Bus Selector6/1
  Logical Operator7/1 -> Bus Creator/4  "OMAPve_y_Prefill_request_1"
  Bus Selector5/11 -> Compare To Constant4/1, Compare To Constant8/1, Switch9/1  "<AEBSve_d_MDDdecRequest_convert>"
  Bus Selector6/6 -> Logical Operator8/2  "<JABSve_d_DbHapticAlarm_convert>"
  Bus Creator/1 -> Out1/1
  Switch6/1 -> Bus Creator1/4, Data Type Conversion10/1  "OMAPve_y_AEB_Braking_progress_1"
  Bus Selector6/3 -> Compare To Constant5/1, Switch6/3, Switch9/3  "<JABSve_d_DbMDDdecRequest_convert>"
  Relational Operator/1 -> Switch3/2, Switch6/2, Switch9/2, Switch10/2
  Logical Operator2/1 -> Logical Operator/2
  Bus Selector5/10 -> Switch6/1  "<AEBSve_d_Braking_progress_convert>"
  Data Type Conversion10/1 -> Bus Creator1/5  "OMAPve_y_Decel_Request_1"
  Bus Selector5/12 -> Compare To Constant3/1, Compare To Constant7/1, Relational Operator/1, Switch10/1  "<AEBSve_g_DecSetpoint_convert>"
  Bus Selector5/9 -> Switch3/1  "<AEBSve_d_MDDdecType_convert>"
  AEB/JA_arb_ELK/1(Out1) -> Bus Creator/5  "OMAPve_y_Haptic_Alarm_1"
  Bus Creator1/1 -> Out2/1
  Bus Selector5/6 -> Logical Operator8/1  "<AEBSve_d_HapticAlarm_convert>"
  Input_AEBS/1 -> Bus Selector5/1
  Bus Selector6/2 -> Switch3/3  "<JABSve_d_DbMDDdecType_convert>"
  Bus Selector6/4 -> Logical Operator7/2  "<JABSve_d_DbPrefillReq_convert>"
  Bus Selector5/4 -> Logical Operator7/1  "<AEBSve_d_Prefill_request_convert>"
  Logical Operator/1 -> Out3/1
  Compare To Constant8/1 -> Logical Operator5/2
  Compare To Constant7/1 -> Logical Operator5/1
  Logical Operator5/1 -> Out4/1
  Compare To Constant5/1 -> Logical Operator/1
  Compare To Constant3/1 -> Logical Operator2/1
  Compare To Constant4/1 -> Logical Operator2/2
  AEB_arb_JA_STATUS/2(Out2) -> Bus Creator/2, Data Type Conversion9/1  "OMAPve_y_State_of_the_functionFARC_det_1"
  Data Type Conversion9/1 -> Bus Creator/3  "OMAPve_y_AEB_Status_1"
  AEB_arb_JA_STATUS/1(Out1) -> Bus Creator/1  "OMAPve_y_FCW_Status_1"
  Bus Selector5/1 -> AEB_arb_JA_STATUS/3(<AEBSve_d_FCWStatus_convert>)  "<AEBSve_d_FCWStatus_convert>"
  Bus Selector5/2 -> AEB_arb_JA_STATUS/4(<AEBSve_d_functionFARCState_convert>)  "<AEBSve_d_functionFARCState_convert>"
  Bus Selector6/9 -> AEB_arb_JA_STATUS/1(<JABSve_d_DbFunFARCSta_convert>)  "<JABSve_d_DbFunFARCSta_convert>"
  Bus Selector6/10 -> AEB_arb_JA_STATUS/2(<JABSve_d_DbJACWStatus_convert>)  "<JABSve_d_DbJACWStatus_convert>"
  Input_ELKS/1 -> AEB/JA_arb_ELK/1(Input_ELKS)
  Logical Operator8/1 -> AEB/JA_arb_ELK/4(AEB+JA_Haptic)
  Bus Selector5/5 -> AEB/JA_arb_ELK/2(AEB_Alert)  "<AEBSve_d_AEBAlertReq_convert>"
  Bus Selector6/5 -> AEB/JA_arb_ELK/3(JA_Alert)  "<JABSve_d_DbAlertReq_convert>"
  Data Type Conversion2/1 -> Bus Creator1/2  "OMAPve_y_ADAS_ESCHoldReq"
  Data Type Conversion1/1 -> Bus Creator1/1  "OMAPve_y_ADAS_ESCDriveOff"
  Bus Selector5/7 -> Logical Operator1/1  "<AEBSve_d_ESCDriveOff_convert>"
  Bus Selector5/8 -> Logical Operator9/1  "<AEBSve_d_ESCHoldReq_convert>"
  Logical Operator1/1 -> Data Type Conversion1/1
  Logical Operator9/1 -> Data Type Conversion2/1
  OMAPve_y_ADAS_ACCRequestEPBNum/1 -> Bus Creator1/8  "OMAPve_y_ADAS_ACCRequestEPB"
  Bus Selector6/7 -> Logical Operator1/2  "<JABSve_d_DbESCDriveOff_convert>"
  Bus Selector6/8 -> Logical Operator9/2  "<JABSve_d_DbESCHoldReq_convert>"
  Switch3/1 -> Bus Creator1/3, [ob_AEBarbJADecType]  "OMAPve_y_MDD_deceleration_type_1"
  Switch10/1 -> [ob_AEBarbJADecSet], Bus Creator1/7  "OMAPve_g_Deceleration_setpoint_device_1"
  Switch9/1 -> [ob_AEBarbJADecReq], Bus Creator1/6  "OMAPve_y_MDD_Decelerationcontrol_request_1"

== system OMAP/Runnable_OMAP_10ms_sys/OMAP_Module/Subsystem/IC_Arbitration/AEB_arb_JA/Subsystem ==
  note: 仲裁#22——AEB/FCW与JAEB/JACW
      | alert优先级：AEB > JAEB > JACW > FCW。若新出现了更高优先级的，则随时覆盖；被覆盖的更低优先级的，不再另计时
  <AEBSve_d_AEBAlertReq_convert> : Inport
  <JABSve_d_DbAlertReq_convert> : Inport  Port=2
  Compare To Constant1 : simulink/Logic and Bit Operations/Compare To Constant  relop===  const=3  OutDataTypeStr=boolean
  Compare To Constant2 : simulink/Logic and Bit Operations/Compare To Constant  relop===  const=3  OutDataTypeStr=boolean
  Compare To Constant3 : simulink/Logic and Bit Operations/Compare To Constant  relop===  const=1  OutDataTypeStr=boolean
  Compare To Constant5 : simulink/Logic and Bit Operations/Compare To Constant  relop===  const=2  OutDataTypeStr=boolean
  Constant : Constant  Value=0  OutDataTypeStr=uint8
  Switch{,1..3} (4 alike) : Switch  Criteria=u2 ~= 0  OutDataTypeStr=uint8
  Out1 : Outport
  wires:
  Switch/1 -> Out1/1
  Compare To Constant5/1 -> Switch/2
  <AEBSve_d_AEBAlertReq_convert>/1 -> Compare To Constant3/1, Switch3/1, Switch/1, Compare To Constant5/1
  Switch1/1 -> Switch/3
  <JABSve_d_DbAlertReq_convert>/1 -> Switch1/1, Compare To Constant1/1, Switch2/1, Compare To Constant2/1
  Compare To Constant1/1 -> Switch1/2
  Switch2/1 -> Switch1/3
  Compare To Constant2/1 -> Switch2/2
  Switch3/1 -> Switch2/3
  Compare To Constant3/1 -> Switch3/2
  Constant/1 -> Switch3/3

== system OMAP/Runnable_OMAP_10ms_sys/OMAP_Module/Subsystem/IC_Arbitration/LKA_arb_ELK/Subsystem ==
  <LKASve_y_EPS_State_Control_convert> : Inport
  <OMAPve_y_General_state_of_LKA_function3F2_2> : Inport  Port=2
  Chart1 : Stateflow chart  TreatAsAtomicUnit=on
  Constant : Constant  Value=OMAP_clb_LKAorELK_CoolTime  OutDataTypeStr=single
  Subsystem1 : Subsystem
  state : Outport
  wires:
  Subsystem1/5(ELK_Down) -> Chart1/5(ELK_Down)
  Subsystem1/6(ELK_Active) -> Chart1/6(ELK_Active)
  Subsystem1/4(ELK_Up) -> Chart1/4(ELK_Up)
  <LKASve_y_EPS_State_Control_convert>/1 -> Subsystem1/1(LKA_State)
  Subsystem1/2(LKA_Down) -> Chart1/2(LKA_Down)
  <OMAPve_y_General_state_of_LKA_function3F2_2>/1 -> Subsystem1/2(ELK_State)
  Constant/1 -> Chart1/7(cool_time)
  Subsystem1/3(LKA_Active) -> Chart1/3(LKA_Active)
  Chart1/1(state) -> state/1
  Subsystem1/1(LKA_Up) -> Chart1/1(LKA_Up)

== system OMAP/Runnable_OMAP_10ms_sys/OMAP_Module/ACCS_Direct/ACCS_Define/ACC_State_Synthesis(ACC_SS)/If Action Subsystem2/Subsystem ==
  In1 : Inport
  Add : Sum  Inputs=+++  OutDataTypeStr=uint8
  Compare To Constant1 : simulink/Logic and Bit Operations/Compare To Constant  relop===  const=0  OutDataTypeStr=boolean
  Compare To Constant2 : simulink/Logic and Bit Operations/Compare To Constant  relop===  const=1  OutDataTypeStr=boolean
  Compare To Constant3 : simulink/Logic and Bit Operations/Compare To Constant  relop===  const=15  OutDataTypeStr=boolean
  Compare To Constant5 : simulink/Logic and Bit Operations/Compare To Constant  relop===  const=2  OutDataTypeStr=boolean
  Compare To Constant6 : simulink/Logic and Bit Operations/Compare To Constant  relop===  const=3  OutDataTypeStr=boolean
  Gain : Gain  Gain=3
  Gain1 : Gain  Gain=2
  Gain2 : Gain  Gain=15
  Logical Operator1 : Logic  Operator=OR  Inputs=3  AllPortsSameDT=off  OutDataTypeStr=boolean
  Function_Acc_status : Outport
  wires:
  Gain2/1 -> Add/3
  Compare To Constant3/1 -> Gain2/1
  Add/1 -> Function_Acc_status/1
  Gain/1 -> Add/1
  Compare To Constant1/1 -> Logical Operator1/1
  Compare To Constant5/1 -> Gain1/1
  Gain1/1 -> Add/2
  Compare To Constant6/1 -> Logical Operator1/3
  In1/1 -> Compare To Constant2/1, Compare To Constant1/1, Compare To Constant6/1, Compare To Constant5/1, Compare To Constant3/1
  Logical Operator1/1 -> Gain/1
  Compare To Constant2/1 -> Logical Operator1/2

== system OMAP/Runnable_OMAP_10ms_sys/OMAP_Module/ACCS_Direct/ACCS_Define/ACC_State_Synthesis(ACC_SS)/If Action Subsystem2/Subsystem4 ==
  Chart : Stateflow chart  TreatAsAtomicUnit=on
  TYPE_RAPPORT : Outport
  wires:
  Chart/1(RAPPORT) -> TYPE_RAPPORT/1

== system OMAP/Runnable_OMAP_10ms_sys/OMAP_Module/ACCS_Direct/ACCS_Define/ACC_State_Synthesis(ACC_SS)/If Action Subsystem3/Subsystem ==
  In1 : Inport
  Constant1 : Constant  Value=6.2  OutDataTypeStr=single
  Constant11 : Constant  Value=6.2  OutDataTypeStr=single
  Switch : Switch  Criteria=u2 > Threshold
  TminDownGear : Outport
  wires:
  Switch/1 -> TminDownGear/1
  Constant1/1 -> Switch/1
  Constant11/1 -> Switch/3
  In1/1 -> Switch/2

== system OMAP/Runnable_OMAP_10ms_sys/OMAP_Module/ACCS_Direct/ACCS_Define/ACC_State_Synthesis(ACC_SS)/If Action Subsystem3/Subsystem1 ==
  In1 : Inport
  Constant12 : Constant  Value=6.2  OutDataTypeStr=single
  Constant2 : Constant  Value=6.2  OutDataTypeStr=single
  Switch1 : Switch  Criteria=u2 > Threshold
  TminUpGear : Outport
  wires:
  Switch1/1 -> TminUpGear/1
  In1/1 -> Switch1/2
  Constant2/1 -> Switch1/1
  Constant12/1 -> Switch1/3

== system OMAP/Runnable_OMAP_10ms_sys/OMAP_Module/ACCS_Direct/ACCS_Define/ACC_State_Synthesis(ACC_SS)/If Action Subsystem3/Subsystem2 ==
  In1 : Inport
  In2 : Inport  Port=2
  Constant1 : Constant  Value=2  OutDataTypeStr=uint8
  Constant11 : Constant  OutDataTypeStr=uint8
  Constant2 : Constant  Value=0  OutDataTypeStr=uint8
  Switch : Switch  Criteria=u2 > Threshold
  Switch1 : Switch  Criteria=u2 > Threshold
  StAcvTqWhlPTPotReq : Outport
  wires:
  In1/1 -> Switch1/2
  In2/1 -> Switch/2
  Constant1/1 -> Switch/1
  Constant2/1 -> Switch/3
  Constant11/1 -> Switch1/1
  Switch/1 -> Switch1/3
  Switch1/1 -> StAcvTqWhlPTPotReq/1

== system OMAP/Runnable_OMAP_10ms_sys/OMAP_Module/ACCS_Direct/ACCS_Define/ACC_State_Synthesis(ACC_SS)/If Action Subsystem3/Subsystem3 ==
  In1 : Inport
  Compare To Constant1 : simulink/Logic and Bit Operations/Compare To Constant  relop===  const=8  OutDataTypeStr=boolean
  Compare To Constant2 : simulink/Logic and Bit Operations/Compare To Constant  relop===  const=7  OutDataTypeStr=boolean
  Constant1 : Constant  Value=7  OutDataTypeStr=uint8
  Logical Operator1 : Logic  Operator=OR  AllPortsSameDT=off  OutDataTypeStr=boolean
  Switch : Switch  Criteria=u2 > Threshold
  Function_Acc_status : Outport
  wires:
  Logical Operator1/1 -> Switch/2
  Switch/1 -> Function_Acc_status/1
  In1/1 -> Switch/3, Compare To Constant1/1, Compare To Constant2/1
  Compare To Constant1/1 -> Logical Operator1/2
  Compare To Constant2/1 -> Logical Operator1/1
  Constant1/1 -> Switch/1

== system OMAP/Runnable_OMAP_10ms_sys/OMAP_Module/ACCS_Direct/ACCS_Define/ACC_State_Synthesis(ACC_SS)/If Action Subsystem3/Subsystem5 ==
  In1 : Inport
  In2 : Inport  Port=2
  Constant4 : Constant  Value=-4000  OutDataTypeStr=single
  Switch : Switch  Criteria=u2 > Threshold
  PotACCTqReq : Outport
  wires:
  In2/1 -> Switch/2
  In1/1 -> Switch/1
  Constant4/1 -> Switch/3
  Switch/1 -> PotACCTqReq/1

== system OMAP/Runnable_OMAP_10ms_sys/OMAP_Module/ACCS_Direct/ACCS_Define/ACC_State_Synthesis(ACC_SS)/If Action Subsystem3/Subsystem6 ==
  Chart : Stateflow chart  TreatAsAtomicUnit=on
  TYPE_RAPPORT : Outport
  wires:
  Chart/1(RAPPORT) -> TYPE_RAPPORT/1

== system OMAP/Runnable_OMAP_10ms_sys/OMAP_Module/ACCS_Direct/ACCS_Define/Human_Machine_Interface(ACC_HMI)/Subsystem9/Subsystem ==
  Bus Creator : BusCreator  Inputs=4
  Constant{,1..3} (4 alike) : Constant  Value=0  OutDataTypeStr=uint16
  Out1 : Outport
  wires:
  Constant/1 -> Bus Creator/1  "ACC_Vehicle_Icon_Display"
  Constant1/1 -> Bus Creator/2  "ACC_Set_Speed_Display"
  Bus Creator/1 -> Out1/1
  Constant2/1 -> Bus Creator/4  "RVVACC_Vehiclespeed_request_type"
  Constant3/1 -> Bus Creator/3  "ACC_DesiredHeadway_Icon_Basic"

== system OMAP/Runnable_OMAP_10ms_sys/OMAP_Module/ACCS_Direct/ACCS_Define/Human_Machine_Interface(ACC_HMI)/Subsystem9/Subsystem1 ==
  VelocitySet : Inport
  Bus Creator : BusCreator  Inputs=4
  Compare To Constant : simulink/Logic and Bit Operations/Compare To Constant  relop=>  const=10  OutDataTypeStr=boolean
  Constant : Constant  OutDataTypeStr=uint16
  Constant2 : Constant  Value=0  OutDataTypeStr=uint16
  Constant3 : Constant  OutDataTypeStr=uint16
  Constant4 : Constant  OutDataTypeStr=uint16
  Constant5 : Constant  Value=3  OutDataTypeStr=uint16
  Switch : Switch
  Out1 : Outport
  wires:
  Constant3/1 -> Bus Creator/3  "ACC_DesiredHeadway_Icon_Basic"
  Constant2/1 -> Bus Creator/4  "RVVACC_Vehiclespeed_request_type"
  Bus Creator/1 -> Out1/1
  Switch/1 -> Bus Creator/2  "ACC_Set_Speed_Display"
  Constant/1 -> Bus Creator/1  "ACC_Vehicle_Icon_Display"
  VelocitySet/1 -> Compare To Constant/1
  Compare To Constant/1 -> Switch/2
  Constant4/1 -> Switch/1
  Constant5/1 -> Switch/3

== system OMAP/Runnable_OMAP_10ms_sys/OMAP_Module/ACCS_Direct/ACCS_Define/Human_Machine_Interface(ACC_HMI)/Subsystem9/Subsystem2 ==
  VelocitySet : Inport
  Bus Creator : BusCreator  Inputs=4
  Compare To Constant : simulink/Logic and Bit Operations/Compare To Constant  relop=>  const=10  OutDataTypeStr=boolean
  Constant : Constant  OutDataTypeStr=uint16
  Constant2 : Constant  Value=0  OutDataTypeStr=uint16
  Constant3 : Constant  OutDataTypeStr=uint16
  Constant4 : Constant  Value=2  OutDataTypeStr=uint16
  Constant5 : Constant  Value=3  OutDataTypeStr=uint16
  Switch : Switch
  Out1 : Outport
  wires:
  Constant/1 -> Bus Creator/1  "ACC_Vehicle_Icon_Display"
  Switch/1 -> Bus Creator/2  "ACC_Set_Speed_Display"
  Bus Creator/1 -> Out1/1
  Constant2/1 -> Bus Creator/4  "RVVACC_Vehiclespeed_request_type"
  Constant3/1 -> Bus Creator/3  "ACC_DesiredHeadway_Icon_Basic"
  VelocitySet/1 -> Compare To Constant/1
  Compare To Constant/1 -> Switch/2
  Constant4/1 -> Switch/1
  Constant5/1 -> Switch/3

== system OMAP/Runnable_OMAP_10ms_sys/OMAP_Module/ACCS_Direct/ACCS_Define/Human_Machine_Interface(ACC_HMI)/Subsystem9/Subsystem3 ==
  Bus Creator : BusCreator  Inputs=4
  Constant : Constant  Value=2  OutDataTypeStr=uint16
  Constant1 : Constant  Value=2  OutDataTypeStr=uint16
  Constant2 : Constant  OutDataTypeStr=uint16
  Constant3 : Constant  OutDataTypeStr=uint16
  Out1 : Outport
  wires:
  Constant3/1 -> Bus Creator/3  "ACC_DesiredHeadway_Icon_Basic"
  Constant2/1 -> Bus Creator/4  "RVVACC_Vehiclespeed_request_type"
  Bus Creator/1 -> Out1/1
  Constant1/1 -> Bus Creator/2  "ACC_Set_Speed_Display"
  Constant/1 -> Bus Creator/1  "ACC_Vehicle_Icon_Display"

== system OMAP/Runnable_OMAP_10ms_sys/OMAP_Module/ACCS_Direct/ACCS_Define/Human_Machine_Interface(ACC_HMI)/Subsystem9/Subsystem4 ==
  Bus Creator : BusCreator  Inputs=4
  Constant : Constant  Value=2  OutDataTypeStr=uint16
  Constant1 : Constant  Value=4  OutDataTypeStr=uint16
  Constant2 : Constant  OutDataTypeStr=uint16
  Constant3 : Constant  OutDataTypeStr=uint16
  Out1 : Outport
  wires:
  Constant/1 -> Bus Creator/1  "ACC_Vehicle_Icon_Display"
  Constant1/1 -> Bus Creator/2  "ACC_Set_Speed_Display"
  Bus Creator/1 -> Out1/1
  Constant2/1 -> Bus Creator/4  "RVVACC_Vehiclespeed_request_type"
  Constant3/1 -> Bus Creator/3  "ACC_DesiredHeadway_Icon_Basic"

== system OMAP/Runnable_OMAP_10ms_sys/OMAP_Module/ACCS_Direct/ACCS_Define/Human_Machine_Interface(ACC_HMI)/Subsystem9/Subsystem5 ==
  Bus Creator : BusCreator  Inputs=4
  Constant : Constant  Value=2  OutDataTypeStr=uint16
  Constant1 : Constant  Value=2  OutDataTypeStr=uint16
  Constant2 : Constant  OutDataTypeStr=uint16
  Constant3 : Constant  OutDataTypeStr=uint16
  Out1 : Outport
  wires:
  Constant3/1 -> Bus Creator/3  "ACC_DesiredHeadway_Icon_Basic"
  Constant2/1 -> Bus Creator/4  "RVVACC_Vehiclespeed_request_type"
  Bus Creator/1 -> Out1/1
  Constant1/1 -> Bus Creator/2  "ACC_Set_Speed_Display"
  Constant/1 -> Bus Creator/1  "ACC_Vehicle_Icon_Display"

== system OMAP/Runnable_OMAP_10ms_sys/OMAP_Module/ACCS_Direct/ACCS_Define/Human_Machine_Interface(ACC_HMI)/Subsystem9/Subsystem6 ==
  Bus Creator : BusCreator  Inputs=4
  Constant : Constant  Value=2  OutDataTypeStr=uint16
  Constant1 : Constant  Value=2  OutDataTypeStr=uint16
  Constant2 : Constant  Value=0  OutDataTypeStr=uint16
  Constant3 : Constant  OutDataTypeStr=uint16
  Out1 : Outport
  wires:
  Constant/1 -> Bus Creator/1  "ACC_Vehicle_Icon_Display"
  Constant1/1 -> Bus Creator/2  "ACC_Set_Speed_Display"
  Bus Creator/1 -> Out1/1
  Constant2/1 -> Bus Creator/4  "RVVACC_Vehiclespeed_request_type"
  Constant3/1 -> Bus Creator/3  "ACC_DesiredHeadway_Icon_Basic"

== system OMAP/Runnable_OMAP_10ms_sys/OMAP_Module/ACCS_Direct/ACCS_Define/Human_Machine_Interface(ACC_HMI)/Subsystem9/Subsystem7 ==
  Bus Creator : BusCreator  Inputs=4
  Constant : Constant  Value=2  OutDataTypeStr=uint16
  Constant1 : Constant  Value=2  OutDataTypeStr=uint16
  Constant2 : Constant  Value=0  OutDataTypeStr=uint16
  Constant3 : Constant  OutDataTypeStr=uint16
  Out1 : Outport
  wires:
  Constant3/1 -> Bus Creator/3  "ACC_DesiredHeadway_Icon_Basic"
  Constant2/1 -> Bus Creator/4  "RVVACC_Vehiclespeed_request_type"
  Bus Creator/1 -> Out1/1
  Constant1/1 -> Bus Creator/2  "ACC_Set_Speed_Display"
  Constant/1 -> Bus Creator/1  "ACC_Vehicle_Icon_Display"

== system OMAP/Runnable_OMAP_10ms_sys/OMAP_Module/ACCS_Direct/ACCS_Define/Human_Machine_Interface(ACC_HMI)/Subsystem9/Subsystem8 ==
  Bus Creator : BusCreator  Inputs=4
  Constant : Constant  Value=3  OutDataTypeStr=uint16
  Constant1 : Constant  Value=3  OutDataTypeStr=uint16
  Constant2 : Constant  Value=0  OutDataTypeStr=uint16
  Constant3 : Constant  Value=0  OutDataTypeStr=uint16
  Out1 : Outport
  wires:
  Constant/1 -> Bus Creator/1  "ACC_Vehicle_Icon_Display"
  Constant1/1 -> Bus Creator/2  "ACC_Set_Speed_Display"
  Bus Creator/1 -> Out1/1
  Constant2/1 -> Bus Creator/4  "RVVACC_Vehiclespeed_request_type"
  Constant3/1 -> Bus Creator/3  "ACC_DesiredHeadway_Icon_Basic"

== system OMAP/Runnable_OMAP_10ms_sys/OMAP_Module/ACCS_Direct/ACCS_Define/Human_Machine_Interface(ACC_HMI)/Text_PopUp/ Radar_Blocked ==
  In1 : Inport
  Chart : Stateflow chart  TreatAsAtomicUnit=on
  Compare To Constant1 : simulink/Logic and Bit Operations/Compare To Constant  relop=~=  const=6  OutDataTypeStr=boolean
  Compare To Constant15 : simulink/Logic and Bit Operations/Compare To Constant  relop===  const=6  OutDataTypeStr=boolean
  Logical Operator : Logic  AllPortsSameDT=off  OutDataTypeStr=boolean
  Unit Delay : UnitDelay  SampleTime=-1
  Out1 : Outport
  wires:
  In1/1 -> Compare To Constant15/1, Unit Delay/1
  Compare To Constant15/1 -> Logical Operator/2
  Unit Delay/1 -> Compare To Constant1/1
  Compare To Constant1/1 -> Logical Operator/1
  Logical Operator/1 -> Chart/1(data)
  Chart/1(Value) -> Out1/1

== system OMAP/Runnable_OMAP_10ms_sys/OMAP_Module/ACCS_Direct/ACCS_Define/Human_Machine_Interface(ACC_HMI)/Text_PopUp/ACC_Activation_Unsatisfied ==
  In1 : Inport
  In2 : Inport  Port=2
  Chart : Stateflow chart  TreatAsAtomicUnit=on
  Compare To Constant17 : simulink/Logic and Bit Operations/Compare To Constant  relop===  const=2  OutDataTypeStr=boolean
  Logical Operator8 : Logic  AllPortsSameDT=off  OutDataTypeStr=boolean
  Out1 : Outport
  wires:
  Compare To Constant17/1 -> Logical Operator8/1
  In2/1 -> Logical Operator8/2
  Logical Operator8/1 -> Chart/1(data)
  In1/1 -> Compare To Constant17/1
  Chart/1(Value) -> Out1/1

== system OMAP/Runnable_OMAP_10ms_sys/OMAP_Module/ACCS_Direct/ACCS_Define/Human_Machine_Interface(ACC_HMI)/Text_PopUp/ACC_Active ==
  In1 : Inport
  Chart : Stateflow chart  TreatAsAtomicUnit=on
  Compare To Constant12 : simulink/Logic and Bit Operations/Compare To Constant  relop===  const=3  OutDataTypeStr=boolean
  Compare To Constant13 : simulink/Logic and Bit Operations/Compare To Constant  relop===  const=4  OutDataTypeStr=boolean
  Logical Operator6 : Logic  AllPortsSameDT=off  OutDataTypeStr=boolean
  Unit Delay1 : UnitDelay  SampleTime=-1
  Out1 : Outport
  wires:
  Unit Delay1/1 -> Compare To Constant12/1
  In1/1 -> Unit Delay1/1, Compare To Constant13/1
  Compare To Constant12/1 -> Logical Operator6/1
  Compare To Constant13/1 -> Logical Operator6/2
  Logical Operator6/1 -> Chart/1(data)
  Chart/1(Value) -> Out1/1
